simulink subsystem "Mach_Controller"  (R2023b)
settings: Solver=VariableStepAuto  StartTime=0.0  StopTime=10.0  RelTol=1e-3
settings Model: Creator=cyber  LastModifiedBy=cyber

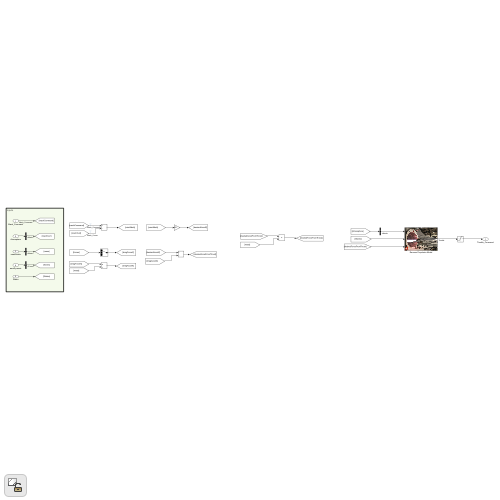
[thumbnail: Simulink's stored preview of the top-level diagram]
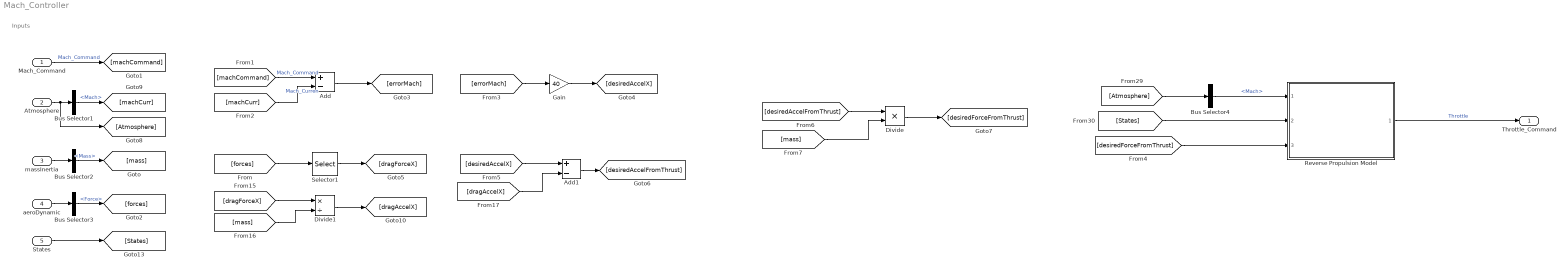
== system Mach_Controller ==
  note: Inputs
  Mach_Command : Inport
  Atmosphere : Inport  Port=2
  massInertia : Inport  Port=3
  aeroDynamic : Inport  Port=4
  States : Inport  Port=5
  Add : Sum  Inputs=+-
  Add1 : Sum  Inputs=+-
  Bus Selector1 : BusSelector  OutputSignals=Mach
  Bus Selector2 : BusSelector  OutputSignals=Mass
  Bus Selector3 : BusSelector  OutputSignals=Force
  Bus Selector4 : BusSelector  OutputSignals=Mach
  Divide : Product  Inputs=**
  Divide1 : Product  Inputs=*/
  Gain : Gain  Gain=40
  Reverse Propulsion Model : Subsystem  ReferencedSubsystem=Reverse_Propulsion_Model
  Selector1 : Selector  InputPortWidth=3  IndexOptions=Index vector (dialog)  Indices=1  OutputSizes=1
  Throttle_Command : Outport
  wires:
  Divide1/1 -> [dragAccelX]
  [mass] -> Divide1/2
  [dragForceX] -> Divide1/1
  States/1 -> [States]
  Divide/1 -> [desiredForceFromThrust]
  [mass] -> Divide/2
  [desiredAccelFromThrust] -> Divide/1
  Add1/1 -> [desiredAccelFromThrust]
  [dragAccelX] -> Add1/2
  [desiredAccelX] -> Add1/1
  Selector1/1 -> [dragForceX]
  Gain/1 -> [desiredAccelX]
  [errorMach] -> Gain/1
  Add/1 -> [errorMach]
  [machCommand] -> Add/1  "Mach_Command"
  [machCurr] -> Add/2  "Mach_Curren"
  [forces] -> Selector1/1
  Bus Selector3/1 -> [forces]  "<Force>"
  aeroDynamic/1 -> Bus Selector3/1
  Bus Selector2/1 -> [mass]  "<Mass>"
  massInertia/1 -> Bus Selector2/1
  Mach_Command/1 -> [machCommand]  "Mach_Command"
  Bus Selector1/1 -> [machCurr]  "<Mach>"
  Atmosphere/1 -> Bus Selector1/1, [Atmosphere]
  [desiredForceFromThrust] -> Reverse Propulsion Model/3
  Reverse Propulsion Model/1 -> Throttle_Command/1  "Throttle"
  [Atmosphere] -> Bus Selector4/1
  [States] -> Reverse Propulsion Model/2
  Bus Selector4/1 -> Reverse Propulsion Model/1  "<Mach>"
